simulink model "part_24"  (R2020a)
settings: Solver=FixedStepAuto  StartTime=0.0  StopTime=1000  FixedStep=0.1  RelTol=1e-3
values from neighbouring files (symbols this model uses):
  A_w = [zeros(3), eye(3) ... (first row only)    [init_NPO.m]
  C_w = [zeros(3) eye(3)]    [init_NPO.m]
  Cur_A_mu = 0.001    [init_current.m]
  Cur_Ac = 0    [init_current.m]
  D = [264860  0  0; 0  881640  0; 0  0  337740000]    [Kalman_data.mat]    (also in init_NPO.m = [2.6486e5  0         0)
  K1 = [diag([K_1i   K_1i   K_1i]) ... (first row only)    [init_NPO.m]
  K2 = K_2i * eye(3)    [init_NPO.m]
  K3 = 0.1*K4    [init_NPO.m]
  K4 = 100000*diag([1 1 100])    [init_NPO.m]
  M_inv = [1.46677031844e-07  0  0; 0  1.2695973473e-07  9.23036390732e-11; 0  9.23036390732e-11  2.80179152408e-10]    [Kalman_data.mat]    (also in init_NPO.m = inv(M))
  OB_mu = 0.001    [init_NPO.m]
  RM_Gamma_matrix = [RM_omega1^2 0 0; 0 RM_omega2^2 0; 0 0 RM_omega3^2]    [init_RM.m]
  RM_Omega_matrix = [2*RM_zeta1*RM_omega1 0 0; 0 2*RM_zeta2*RM_omega2 0; 0 0 2*RM_zeta3*RM_omega3]    [init_RM.m]
  RM_t1 = 15    [init_RM.m]
  RM_t2 = 15    [init_RM.m]
  RM_t3 = 15    [init_RM.m]
  setp_n = 6    [init_RM.m]
  setpoint = [0,0,0 ... (first row only)    [init_RM.m]
  T_b = diag([T_b1 T_b2 T_b3])    [init_NPO.m]
undefined symbols (not defined in the file or in its folder): DP_Kd_matrix, DP_Ki_matrix, DP_Kp_matrix, Hoerner, K, P_0, posX, posY, vessel, Wind_A_mu, Wind_Cw, Wind_mu, x_0
libraries: marine_gnc x9, simulink x5, marine_hydro x2
settings Model: OrderedModelArguments=off  Creator=jonbjor  LastModifiedBy=USER
settings DataIOCC: ReturnWorkspaceOutputs=off
settings DebuggingCC: ArithmeticOperatorsInVariantConditions=warning
settings SFSimCC: SimUseLocalCustomCode=off  CustomCodeUndefinedFunction=UseInterfaceOnly
settings RTWCC: RTWUseLocalCustomCode=off

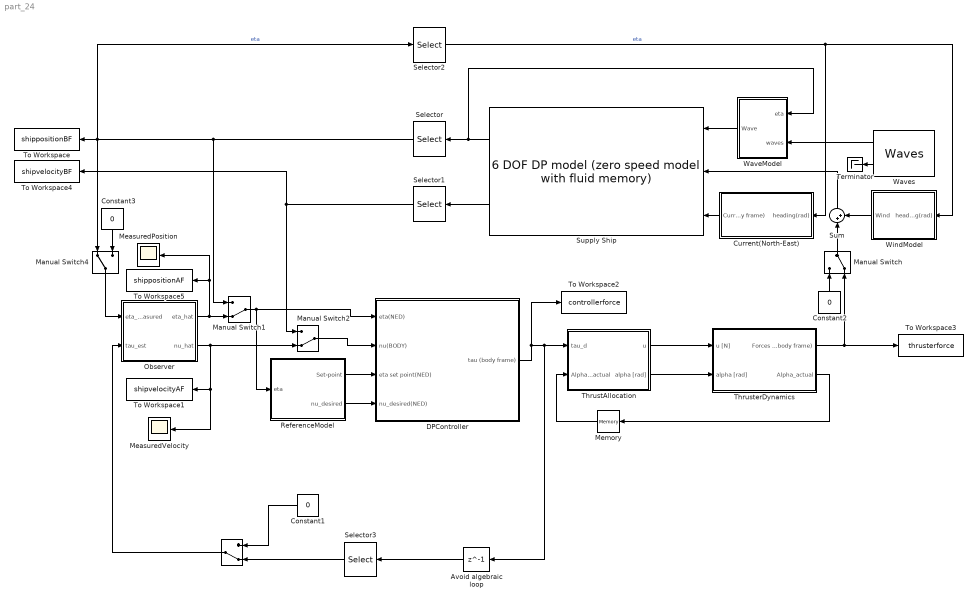
== system part_24 ==
  "\t\t" : ManualSwitch  CurrentSetting=0
  Avoid algebraic loop : Delay  DelayLength=1
  Constant1 : Constant  Value=0  VectorParams1D=off
  Constant2 : Constant  Value=0  VectorParams1D=off
  Constant3 : Constant  Value=0  VectorParams1D=off
  Current(North-East) : Subsystem
  DPController : Subsystem
  Manual Switch : ManualSwitch  CurrentSetting=0
  Manual Switch1 : ManualSwitch  CurrentSetting=0
  Manual Switch2 : ManualSwitch  CurrentSetting=0
  Manual Switch4 : ManualSwitch
  MeasuredPosition : Scope
  MeasuredVelocity : Scope
  Memory : Memory
  Observer : Subsystem
  ReferenceModel : Subsystem
  Selector : Selector  InputPortWidth=6  IndexOptions=Index vector (dialog)  Indices=[1 2 6]  OutputSizes=1
  Selector1 : Selector  InputPortWidth=6  IndexOptions=Index vector (dialog)  Indices=[1 2 6]  OutputSizes=1
  Selector2 : Selector  InputPortWidth=3  IndexOptions=Index vector (dialog)  Indices=[3]  OutputSizes=1
  Selector3 : Selector  InputPortWidth=6  IndexOptions=Index vector (dialog)  Indices=[1 2 6]  OutputSizes=1
  Sum : Sum  Inputs=|++
  Supply Ship : marine_hydro/Hydro Library/6 DOF DP model  (zero speed model with fluid memory)  ABC=vesselABC  rho=1025  Axc=0.9*vessel.main.T*vessel.main.B  Ayc=0.9*vessel.main.T*vessel.main.Lpp  CX=1  CY_2D=Hoerner(vessel.main.B,vessel.main.T)  Bv=vessel.Bv  mask(6 DOF zero speed model){}
      link override "Integrator1 ": InitialCondition=nu0
      link override Integrator2: InitialCondition=eta0
      settings: SourceProductName=MSS Hydro
      mask Display:
      | image('supply.jpg');
      | color('white'); port_label('output', 1, 'eta')
      | color('white'); port_label('output', 2, 'nu')
      | color('white'); port_label('input', 1, 'tau_wave')
      | color('white'); port_label('input', 2, 'tau')
      | color('white'); port_label('input', 3, 'nu_c')
  Terminator : Terminator
  ThrustAllocation : Subsystem
  ThrusterDynamics : Subsystem  mask{thrusterfault=off}
      mask prompts: thrusterfault "Fault on thruster #2 and #5?"
  To Workspace : ToWorkspace  VariableName=shippositionBF  SaveFormat=Structure With Time  SampleTime=-1
  To Workspace1 : ToWorkspace  VariableName=shipvelocityAF  SaveFormat=Structure With Time  SampleTime=-1
  To Workspace2 : ToWorkspace  VariableName=controllerforce  SaveFormat=Structure With Time  SampleTime=-1
  To Workspace3 : ToWorkspace  VariableName=thrusterforce  SaveFormat=Structure With Time  SampleTime=-1
  To Workspace4 : ToWorkspace  VariableName=shipvelocityBF  SaveFormat=Structure With Time  SampleTime=-1
  To Workspace5 : ToWorkspace  VariableName=shippositionAF  SaveFormat=Structure With Time  SampleTime=-1
  WaveModel : Subsystem  mask{waveforces=on}
      mask prompts: waveforces "Waveforces enabled"
  Waves : marine_gnc/Environment/Waves/Waves  spectrum_type=ITTC  disp_flag=on  plot_spectrum=off  plot_realization=off  hs=8  omega_peak=2*pi/13  psi_mean=5*pi/4  gamma=-1  spread=2  depth=inf  nfreq=20  ndir=10  energylim=0.005  freq_cutoff=3  dir_cutoff=0  rand_seed=123  rand_freq=off  rand_dir=off  Zeta_a=0  Omega=0  Phase=0  Wavenum=0  Psi=0
      settings: SourceProductName=MSS GNC
  WindModel : Subsystem
  wires:
  Supply Ship/2 -> Selector1/1
  ReferenceModel/1(Set-point) -> DPController/3(eta set point(NED))
  Supply Ship/1 -> WaveModel/1(eta), Selector/1
  Current(North-East)/1(Current(body frame)) -> Supply Ship/3
  WaveModel/1(Wave) -> Supply Ship/1
  Waves/1 -> WaveModel/2(waves)
  Waves/2 -> Terminator/1
  WindModel/1(Wind) -> Sum/2
  ThrusterDynamics/1("Forces (body frame) ") -> Manual Switch/2, To Workspace3/1
  Selector2/1 -> WindModel/1(heading(rad)), Current(North-East)/1(heading(rad))  "eta"
  ThrustAllocation/1(u) -> ThrusterDynamics/1(u [N])
  ThrustAllocation/2(alpha [rad]) -> ThrusterDynamics/2(alpha [rad])
  ReferenceModel/2(nu_desired) -> DPController/4(nu_desired(NED))
  Sum/1 -> Supply Ship/2
  Manual Switch/1 -> Sum/1
  Constant2/1 -> Manual Switch/1
  Memory/1 -> ThrustAllocation/2(Alpha_actual)
  ThrusterDynamics/2(Alpha_actual) -> Memory/1
  Selector/1 -> Manual Switch1/1, Selector2/1, To Workspace/1, Manual Switch4/1  "eta"
  Observer/2(nu_hat) -> MeasuredVelocity/1, To Workspace1/1, Manual Switch2/2
  Observer/1(eta_hat) -> MeasuredPosition/1, To Workspace5/1, Manual Switch1/2
  "\t\t"/1 -> Observer/2(tau_est)
  Constant1/1 -> "\t\t"/1
  Manual Switch4/1 -> Observer/1(eta_measured)
  Constant3/1 -> Manual Switch4/2
  Avoid algebraic loop/1 -> Selector3/1
  DPController/1(tau (body frame)) -> To Workspace2/1, Avoid algebraic loop/1, ThrustAllocation/1(tau_d)
  Manual Switch1/1 -> DPController/1(eta(NED)), ReferenceModel/1(eta)
  Manual Switch2/1 -> DPController/2(nu(BODY))
  Selector3/1 -> "\t\t"/2
  Selector1/1 -> To Workspace4/1, Manual Switch2/1

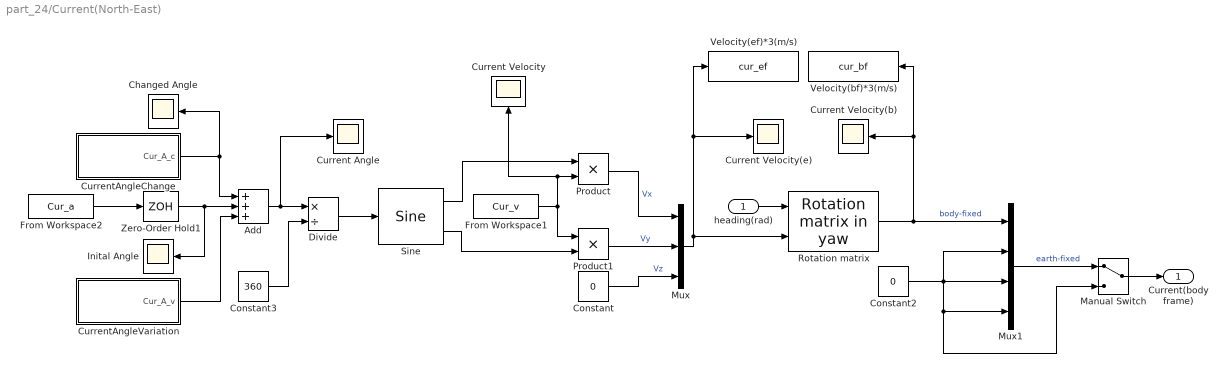
== system part_24/Current(North-East) ==
  heading(rad) : Inport
  Add : Sum  Inputs=+++
  Changed Angle : Scope
  Constant : Constant  Value=0
  Constant2 : Constant  Value=0  VectorParams1D=off
  Constant3 : Constant  Description=It is the angle of the current  Value=360
  Current Angle : Scope
  Current Velocity : Scope
  Current Velocity(b) : Scope
  Current Velocity(e) : Scope
  CurrentAngleChange : Subsystem
  CurrentAngleVariation : Subsystem
  Divide : Product  Inputs=*/
  From Workspace1 : FromWorkspace  VariableName=Cur_v  OutputAfterFinalValue=Holding final value
  From Workspace2 : FromWorkspace  VariableName=Cur_a  OutputAfterFinalValue=Holding final value
  Inital Angle : Scope
  Manual Switch : ManualSwitch
  Mux : Mux  Inputs=3
  Mux1 : Mux
  Product : Product
  Product1 : Product
  "Rotation matrix " : marine_gnc/Models/ Kinematics/Rotation matrix in yaw 
      settings: SourceProductName=MSS GNC
  Sine : simulink/Lookup Tables/Sine  Formula=sin(2*pi*u) and cos(2*pi*u)  NumDataPoints=(2^5)+1  OutputWordLength=16  InternalRulePriority=Speed
  Velocity(bf)*3(m/s) : ToWorkspace  VariableName=cur_bf  SaveFormat=Structure With Time  SampleTime=-1
  Velocity(ef)*3(m/s) : ToWorkspace  VariableName=cur_ef  SaveFormat=Structure With Time  SampleTime=-1
  Zero-Order Hold1 : ZeroOrderHold  SampleTime=-1
  Current(body frame) : Outport  VectorParamsAs1DForOutWhenUnconnected=off
  wires:
  From Workspace2/1 -> Zero-Order Hold1/1
  Sine/1 -> Product/1
  Divide/1 -> Sine/1
  Sine/2 -> Product1/2
  CurrentAngleChange/1(Cur_A_c) -> Add/1, Changed Angle/1
  From Workspace1/1 -> Current Velocity/1, Product/2, Product1/1
  Product/1 -> Mux/1  "Vx"
  Mux/1 -> Velocity(ef)*3(m/s)/1, Current Velocity(e)/1, "Rotation matrix "/2
  heading(rad)/1 -> "Rotation matrix "/1
  Product1/1 -> Mux/2  "Vy"
  "Rotation matrix "/1 -> Velocity(bf)*3(m/s)/1, Current Velocity(b)/1, Mux1/1  "body-fixed"
  Add/1 -> Current Angle/1, Divide/1
  Constant2/1 -> Mux1/2, Manual Switch/2, Mux1/4, Mux1/3
  Constant3/1 -> Divide/2
  Constant/1 -> Mux/3  "Vz"
  Manual Switch/1 -> Current(body frame)/1
  Zero-Order Hold1/1 -> Inital Angle/1, Add/2
  CurrentAngleVariation/1(Cur_A_v) -> Add/3
  Mux1/1 -> Manual Switch/1  "earth-fixed"

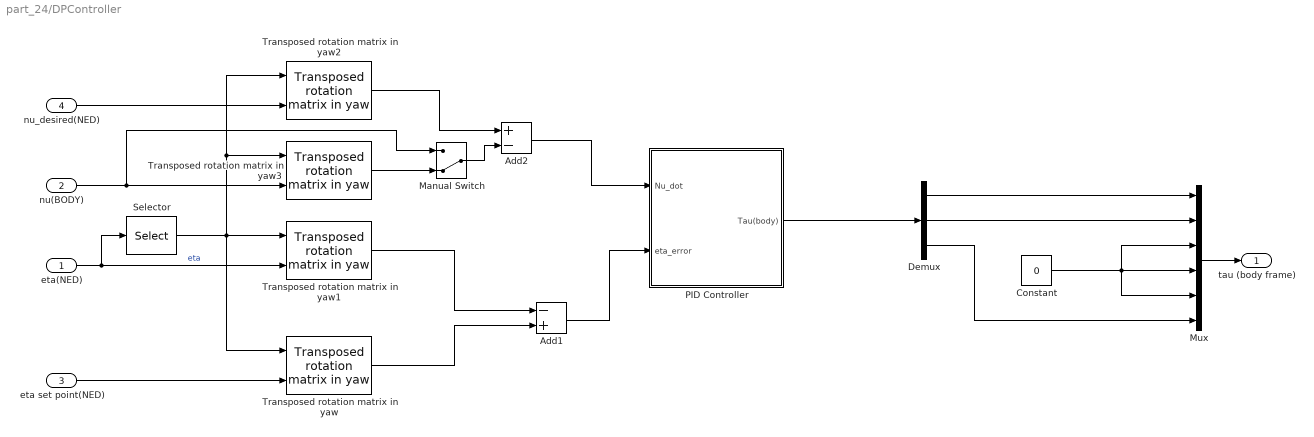
== system part_24/DPController ==
  eta(NED) : Inport
  nu(BODY) : Inport  Port=2
  eta set point(NED) : Inport  Port=3
  nu_desired(NED) : Inport  Port=4
  Add1 : Sum  Inputs=-+
  Add2 : Sum  Inputs=+-
  Constant : Constant  Value=0
  Demux : Demux  Outputs=3
  Manual Switch : ManualSwitch  CurrentSetting=0
  Mux : Mux  Inputs=6
  "PID Controller " : Subsystem
  Selector : Selector  InputPortWidth=3  IndexOptions=Starting index (dialog)  Indices=[3]  OutputSizes=1
  Transposed rotation matrix in yaw{,1..3} (4 alike) : marine_gnc/Models/ Kinematics/Transposed rotation  matrix in yaw
      settings: SourceProductName=MSS GNC
  tau (body frame) : Outport  VectorParamsAs1DForOutWhenUnconnected=off
  wires:
  nu_desired(NED)/1 -> Transposed rotation matrix in yaw2/2
  eta(NED)/1 -> Selector/1, Transposed rotation matrix in yaw1/2  "eta"
  Transposed rotation matrix in yaw1/1 -> Add1/1
  Transposed rotation matrix in yaw/1 -> Add1/2
  Add1/1 -> "PID Controller "/2("eta_error ")
  eta set point(NED)/1 -> Transposed rotation matrix in yaw/2
  "PID Controller "/1(Tau(body)) -> Demux/1
  Selector/1 -> Transposed rotation matrix in yaw3/1, Transposed rotation matrix in yaw2/1, Transposed rotation matrix in yaw/1, Transposed rotation matrix in yaw1/1
  Demux/2 -> Mux/2
  Add2/1 -> "PID Controller "/1("Nu_dot ")
  Demux/1 -> Mux/1
  Mux/1 -> tau (body frame)/1
  Transposed rotation matrix in yaw2/1 -> Add2/1
  Constant/1 -> Mux/5, Mux/4, Mux/3
  Demux/3 -> Mux/6
  Transposed rotation matrix in yaw3/1 -> Manual Switch/2
  Manual Switch/1 -> Add2/2
  nu(BODY)/1 -> Manual Switch/1, Transposed rotation matrix in yaw3/2

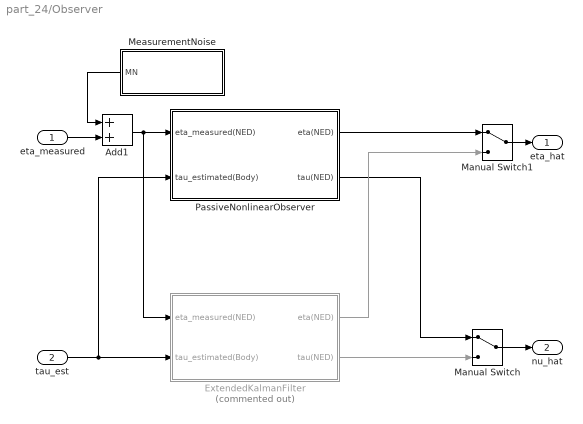
== system part_24/Observer ==
  eta_measured : Inport
  tau_est : Inport  Port=2
  Add1 : Sum
  ExtendedKalmanFilter : Subsystem  Commented=on
  Manual Switch : ManualSwitch
  Manual Switch1 : ManualSwitch
  MeasurementNoise : Subsystem
  PassiveNonlinearObserver : Subsystem
  eta_hat : Outport  VectorParamsAs1DForOutWhenUnconnected=off
  nu_hat : Outport  Port=2  VectorParamsAs1DForOutWhenUnconnected=off
  wires:
  PassiveNonlinearObserver/1(eta(NED)) -> Manual Switch1/1
  PassiveNonlinearObserver/2(tau(NED)) -> Manual Switch/1
  ExtendedKalmanFilter/1(eta(NED)) -> Manual Switch1/2
  ExtendedKalmanFilter/2(tau(NED)) -> Manual Switch/2
  tau_est/1 -> ExtendedKalmanFilter/2(tau_estimated(Body)), PassiveNonlinearObserver/2(tau_estimated(Body))
  Manual Switch/1 -> nu_hat/1
  Manual Switch1/1 -> eta_hat/1
  eta_measured/1 -> Add1/2
  Add1/1 -> ExtendedKalmanFilter/1(eta_measured(NED)), PassiveNonlinearObserver/1(eta_measured(NED))
  MeasurementNoise/1(MN) -> Add1/1

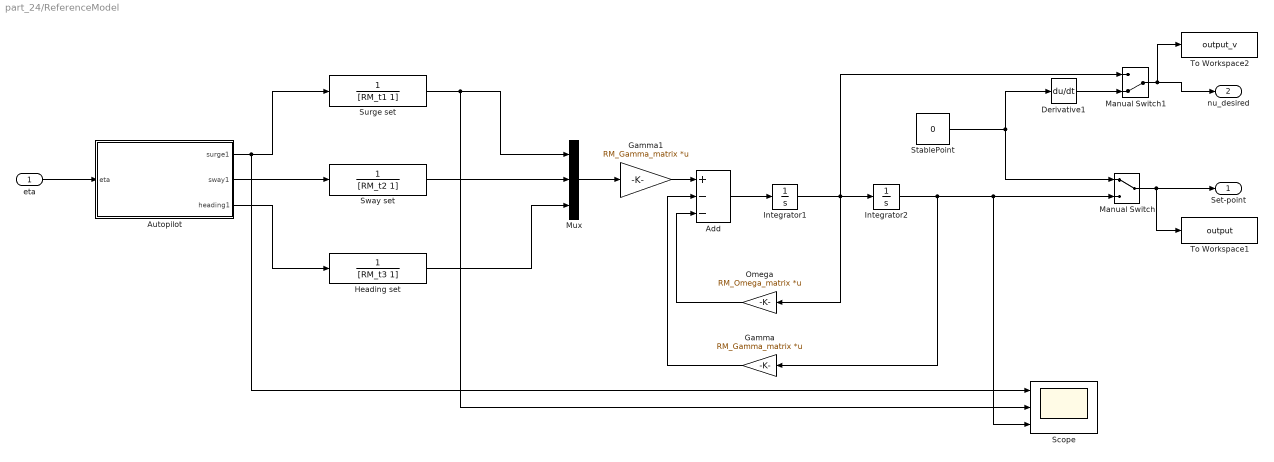
== system part_24/ReferenceModel ==
  eta : Inport
  Add : Sum  Inputs=+--
  Autopilot : Subsystem
  Derivative1 : Derivative
  Gamma : Gain  Gain=RM_Gamma_matrix  Multiplication=Matrix(K*u)
  Gamma1 : Gain  Gain=RM_Gamma_matrix  Multiplication=Matrix(K*u)
  Heading set : TransferFcn  Denominator=[RM_t3 1]
  Integrator1 : Integrator
  Integrator2 : Integrator
  Manual Switch : ManualSwitch
  Manual Switch1 : ManualSwitch  CurrentSetting=0
  Mux : Mux  Inputs=3
  Omega : Gain  Gain=RM_Omega_matrix  Multiplication=Matrix(K*u)
  Scope : Scope  NumInputPorts=3
  StablePoint : Constant  Value=0
  Surge set : TransferFcn  Denominator=[RM_t1 1]
  Sway set : TransferFcn  Denominator=[RM_t2 1]
  To Workspace1 : ToWorkspace  VariableName=output  SaveFormat=Structure With Time  SampleTime=-1
  To Workspace2 : ToWorkspace  VariableName=output_v  SaveFormat=Structure With Time  SampleTime=-1
  Set-point : Outport  VectorParamsAs1DForOutWhenUnconnected=off
  nu_desired : Outport  Port=2
  wires:
  Add/1 -> Integrator1/1
  StablePoint/1 -> Derivative1/1, Manual Switch/1
  Surge set/1 -> Mux/1, Scope/2
  Integrator1/1 -> Manual Switch1/1, Integrator2/1, Omega/1
  Gamma/1 -> Add/2
  Omega/1 -> Add/3
  Integrator2/1 -> Gamma/1, Scope/3, Manual Switch/2
  Heading set/1 -> Mux/3
  Mux/1 -> Gamma1/1
  Sway set/1 -> Mux/2
  Gamma1/1 -> Add/1
  Manual Switch/1 -> Set-point/1, To Workspace1/1
  eta/1 -> Autopilot/1(eta)
  Autopilot/1(surge1) -> Scope/1, Surge set/1
  Autopilot/2(sway1) -> Sway set/1
  Autopilot/3(heading1) -> Heading set/1
  Manual Switch1/1 -> To Workspace2/1, nu_desired/1
  Derivative1/1 -> Manual Switch1/2

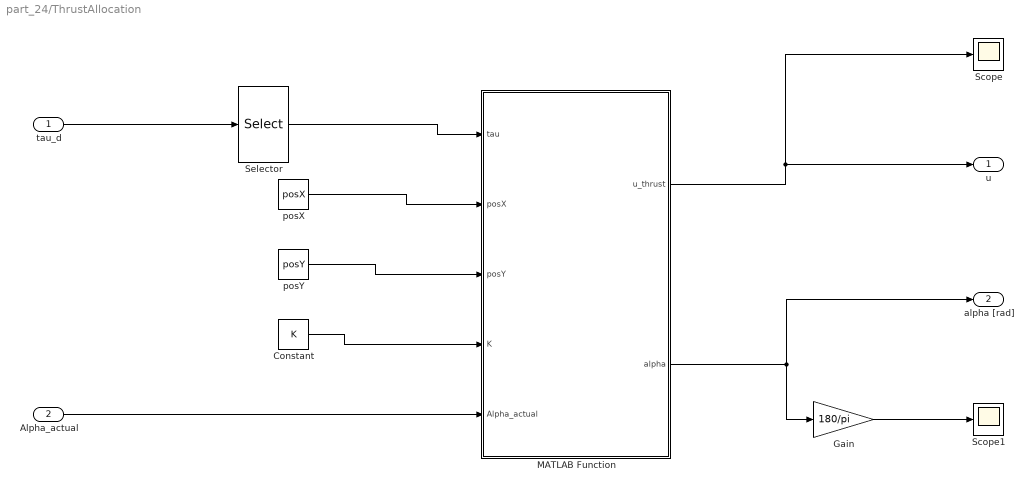
== system part_24/ThrustAllocation ==
  tau_d : Inport
  Alpha_actual : Inport  Port=2
  Constant : Constant  Value=K
  Gain : Gain  Gain=180/pi
  MATLAB Function : MATLAB Function  TreatAsAtomicUnit=on
  Scope : Scope
  Scope1 : Scope
  Selector : Selector  InputPortWidth=6  IndexOptions=Index vector (dialog)  Indices=[1 2 6 ]  OutputSizes=1
  posX : Constant  Value=posX
  posY : Constant  Value=posY
  u : Outport
  alpha [rad] : Outport  Port=2
  wires:
  tau_d/1 -> Selector/1
  MATLAB Function/1(u_thrust) -> Scope/1, u/1
  MATLAB Function/2(alpha) -> alpha [rad]/1, Gain/1
  Selector/1 -> MATLAB Function/1(tau)
  Gain/1 -> Scope1/1
  posX/1 -> MATLAB Function/2(posX)
  posY/1 -> MATLAB Function/3(posY)
  Constant/1 -> MATLAB Function/4(K)
  Alpha_actual/1 -> MATLAB Function/5(Alpha_actual)

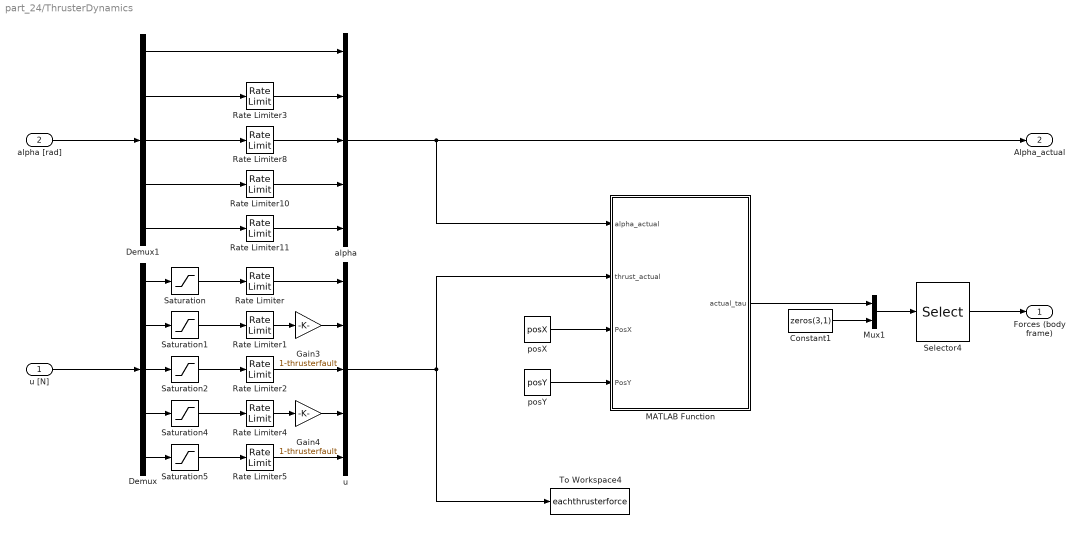
== system part_24/ThrusterDynamics ==
  u [N] : Inport
  alpha [rad] : Inport  Port=2
  Constant1 : Constant  Value=zeros(3,1)
  Demux : Demux  Outputs=5
  Demux1 : Demux  Outputs=5
  Gain3 : Gain  Gain=1-thrusterfault
  Gain4 : Gain  Gain=1-thrusterfault
  MATLAB Function : MATLAB Function  TreatAsAtomicUnit=on
  Mux1 : Mux  Inputs=2
  Rate Limiter : RateLimiter  RisingSlewLimit=15625  FallingSlewLimit=-15625  SampleTimeMode=inherited
  Rate Limiter1 : RateLimiter  RisingSlewLimit=18750  FallingSlewLimit=-18750  SampleTimeMode=inherited
  Rate Limiter{3,8,10..11} (4 alike) : RateLimiter  RisingSlewLimit=pi/15  FallingSlewLimit=-pi/15  SampleTimeMode=inherited
  Rate Limiter2 : RateLimiter  RisingSlewLimit=18750  FallingSlewLimit=-18750  SampleTimeMode=inherited
  Rate Limiter4 : RateLimiter  RisingSlewLimit=32000  FallingSlewLimit=-32000  SampleTimeMode=inherited
  Rate Limiter5 : RateLimiter  RisingSlewLimit=32000  FallingSlewLimit=-32000  SampleTimeMode=inherited
  Saturation : Saturate  UpperLimit=125000  LowerLimit=0
  Saturation1 : Saturate  UpperLimit=150000  LowerLimit=0
  Saturation2 : Saturate  UpperLimit=150000  LowerLimit=0
  Saturation4 : Saturate  UpperLimit=320000  LowerLimit=0
  Saturation5 : Saturate  UpperLimit=320000  LowerLimit=0
  Selector4 : Selector  InputPortWidth=6  IndexOptions=Index vector (dialog)  Indices=[1 2 4 5 6 3]  OutputSizes=1
  To Workspace4 : ToWorkspace  VariableName=eachthrusterforce  SaveFormat=Structure With Time  SampleTime=-1
  alpha : Mux  Inputs=5
  posX : Constant  Value=posX  VectorParams1D=off
  posY : Constant  Value=posY  VectorParams1D=off
  u : Mux  Inputs=5
  "Forces (body frame) " : Outport
  Alpha_actual : Outport  Port=2
  wires:
  Rate Limiter2/1 -> u/3
  Saturation/1 -> Rate Limiter/1
  Mux1/1 -> Selector4/1
  Constant1/1 -> Mux1/2
  Saturation4/1 -> Rate Limiter4/1
  Demux/2 -> Saturation1/1
  Saturation1/1 -> Rate Limiter1/1
  Demux/1 -> Saturation/1
  Demux/3 -> Saturation2/1
  Saturation2/1 -> Rate Limiter2/1
  Selector4/1 -> "Forces (body frame) "/1
  Rate Limiter/1 -> u/1
  Saturation5/1 -> Rate Limiter5/1
  Rate Limiter8/1 -> alpha/3
  u [N]/1 -> Demux/1
  alpha [rad]/1 -> Demux1/1
  posX/1 -> MATLAB Function/3(PosX)
  posY/1 -> MATLAB Function/4(PosY)
  alpha/1 -> Alpha_actual/1, MATLAB Function/1(alpha_actual)
  Demux1/3 -> Rate Limiter8/1
  Rate Limiter10/1 -> alpha/4
  Demux1/4 -> Rate Limiter10/1
  Demux1/5 -> Rate Limiter11/1
  Rate Limiter11/1 -> alpha/5
  Demux1/2 -> Rate Limiter3/1
  Demux1/1 -> alpha/1
  Demux/4 -> Saturation4/1
  Demux/5 -> Saturation5/1
  Rate Limiter5/1 -> u/5
  Rate Limiter3/1 -> alpha/2
  Rate Limiter1/1 -> Gain3/1
  MATLAB Function/1(actual_tau) -> Mux1/1
  u/1 -> To Workspace4/1, MATLAB Function/2(thrust_actual)
  Rate Limiter4/1 -> Gain4/1
  Gain3/1 -> u/2
  Gain4/1 -> u/4

== system part_24/WaveModel ==
  eta : Inport
  waves : Inport  Port=2
  Constant1 : Constant  Value=0  VectorParams1D=off
  Gain : Gain  Gain=waveforces
  Manual Switch1 : ManualSwitch  CurrentSetting=0
  Sum : Sum
  Wave loads (U=0) : marine_hydro/Hydro Library/Wave loads (U=0)  SystemSampleTime=-1  Latency=0  AutoFrameSizeCalculation=off
      settings: SourceProductName=MSS Hydro
  Wave : Outport  VectorParamsAs1DForOutWhenUnconnected=off
  wires:
  eta/1 -> Wave loads (U=0)/1
  waves/1 -> Wave loads (U=0)/2
  Sum/1 -> Gain/1
  Wave loads (U=0)/1 -> Sum/1
  Wave loads (U=0)/2 -> Sum/2
  Constant1/1 -> Manual Switch1/1
  Gain/1 -> Manual Switch1/2
  Manual Switch1/1 -> Wave/1

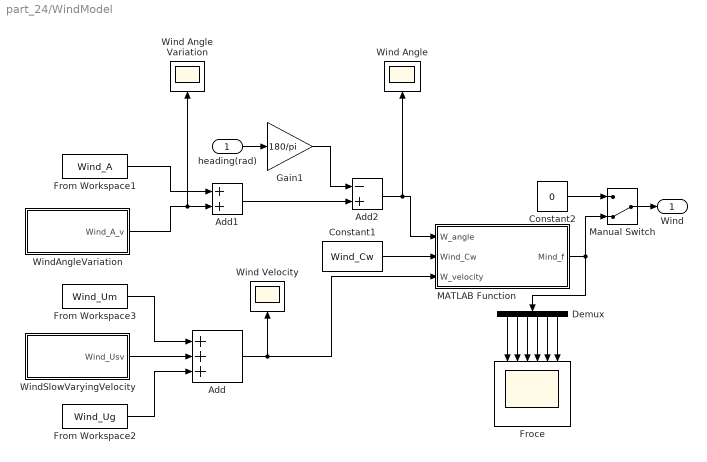
== system part_24/WindModel ==
  heading(rad) : Inport
  Add : Sum  Inputs=+++
  Add1 : Sum
  Add2 : Sum  Inputs=-+
  Constant1 : Constant  Value=Wind_Cw  SampleTime=0
  Constant2 : Constant  Value=0  VectorParams1D=off
  Demux : Demux  Outputs=6
  Froce : Scope  NumInputPorts=6
  From Workspace1 : FromWorkspace  VariableName=Wind_A  OutputAfterFinalValue=Holding final value
  From Workspace2 : FromWorkspace  VariableName=Wind_Ug  OutputAfterFinalValue=Holding final value
  From Workspace3 : FromWorkspace  VariableName=Wind_Um  OutputAfterFinalValue=Holding final value
  Gain1 : Gain  Gain=180/pi
  MATLAB Function : MATLAB Function  TreatAsAtomicUnit=on
  Manual Switch : ManualSwitch  CurrentSetting=0
  Wind Angle : Scope
  Wind Angle Variation : Scope
  Wind Velocity : Scope
  WindAngleVariation : Subsystem
  WindSlowVaryingVelocity : Subsystem
  Wind : Outport  VectorParamsAs1DForOutWhenUnconnected=off
  wires:
  Manual Switch/1 -> Wind/1
  From Workspace3/1 -> Add/1
  WindSlowVaryingVelocity/1(Wind_Usv) -> Add/2
  WindAngleVariation/1(Wind_A_v) -> Wind Angle Variation/1, Add1/2
  From Workspace1/1 -> Add1/1
  heading(rad)/1 -> Gain1/1
  Add1/1 -> Add2/2
  Gain1/1 -> Add2/1
  Add2/1 -> Wind Angle/1, MATLAB Function/1(W_angle)
  MATLAB Function/1(Mind_f) -> Manual Switch/2, Demux/1
  Constant1/1 -> MATLAB Function/2(Wind_Cw)
  Demux/1 -> Froce/1
  Demux/6 -> Froce/6
  Demux/5 -> Froce/5
  Demux/3 -> Froce/3
  Demux/2 -> Froce/2
  Demux/4 -> Froce/4
  Add/1 -> MATLAB Function/3(W_velocity), Wind Velocity/1
  From Workspace2/1 -> Add/3
  Constant2/1 -> Manual Switch/1

== system part_24/Current(North-East)/CurrentAngleChange ==
  Constant4 : Constant  Description=It is the angle of the current  Value=0
  Constant5 : Constant  Value=Cur_Ac
  From Workspace3 : FromWorkspace  VariableName=Cur_ac  SampleTime=0.1  Interpolate=off  OutputAfterFinalValue=Holding final value
  Switch : Switch  Criteria=u2 > Threshold
  Zero-Order Hold : ZeroOrderHold  SampleTime=-1
  Cur_A_c : Outport
  wires:
  Zero-Order Hold/1 -> Switch/1
  Constant5/1 -> Switch/2
  From Workspace3/1 -> Zero-Order Hold/1
  Constant4/1 -> Switch/3
  Switch/1 -> Cur_A_c/1

== system part_24/Current(North-East)/CurrentAngleVariation ==
  Add : Sum  Inputs=+-
  Band-Limited White Noise : simulink/Sources/Band-Limited White Noise  Cov=Cur_A_w  Ts=1  seed=[23341]
  Constant : Constant  Value=Cur_A_mu
  Integrator : Integrator
  prod : Product  Inputs=**
  Cur_A_v : Outport
  wires:
  Integrator/1 -> Cur_A_v/1, prod/2
  Constant/1 -> prod/1
  Band-Limited White Noise/1 -> Add/1
  prod/1 -> Add/2
  Add/1 -> Integrator/1  "Udot"

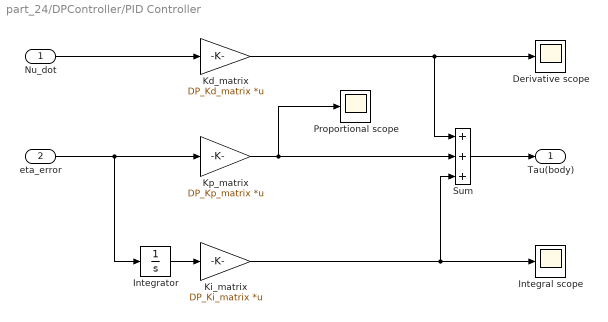
== system part_24/DPController/PID Controller  ==
  "Nu_dot " : Inport
  "eta_error " : Inport  Port=2
  "Derivative scope " : Scope
  "Integral scope " : Scope
  Integrator : Integrator
  "Kd_matrix " : Gain  Gain=DP_Kd_matrix  Multiplication=Matrix(K*u)
  "Ki_matrix " : Gain  Gain=DP_Ki_matrix  Multiplication=Matrix(K*u)
  Kp_matrix : Gain  Gain=DP_Kp_matrix  Multiplication=Matrix(K*u)
  "Proportional scope " : Scope
  Sum : Sum  Inputs=+++
  Tau(body) : Outport  VectorParamsAs1DForOutWhenUnconnected=off
  wires:
  "eta_error "/1 -> Integrator/1, Kp_matrix/1
  "Nu_dot "/1 -> "Kd_matrix "/1
  Integrator/1 -> "Ki_matrix "/1
  Kp_matrix/1 -> "Proportional scope "/1, Sum/2
  "Kd_matrix "/1 -> "Derivative scope "/1, Sum/1
  Sum/1 -> Tau(body)/1
  "Ki_matrix "/1 -> Sum/3, "Integral scope "/1

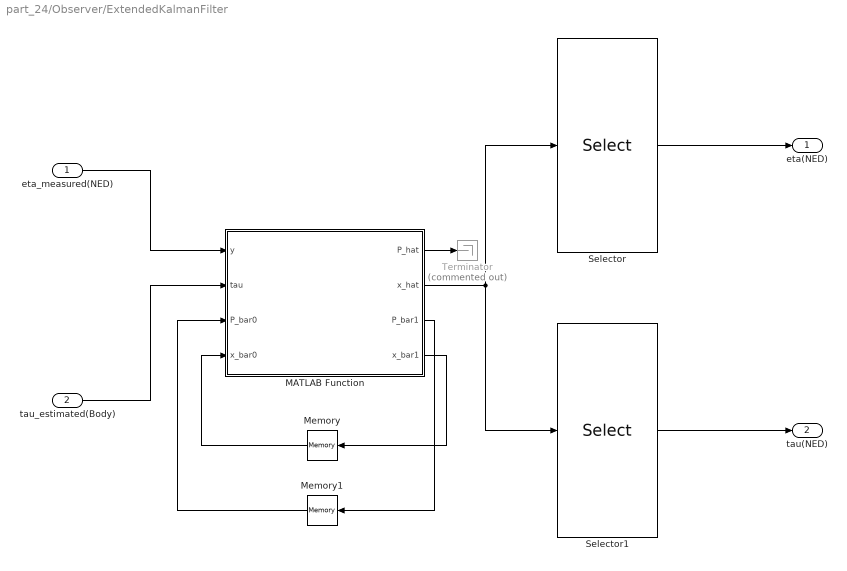
== system part_24/Observer/ExtendedKalmanFilter ==
  eta_measured(NED) : Inport
  tau_estimated(Body) : Inport  Port=2
  MATLAB Function : MATLAB Function  TreatAsAtomicUnit=on
  Memory : Memory  InitialCondition=x_0
  Memory1 : Memory  InitialCondition=P_0
  Selector : Selector  InputPortWidth=15  IndexOptions=Index vector (dialog)  Indices=[7 8 9]  OutputSizes=1
  Selector1 : Selector  InputPortWidth=15  IndexOptions=Index vector (dialog)  Indices=[13 14 15]  OutputSizes=1
  Terminator : Terminator  Commented=on
  eta(NED) : Outport
  tau(NED) : Outport  Port=2
  wires:
  eta_measured(NED)/1 -> MATLAB Function/1(y)
  tau_estimated(Body)/1 -> MATLAB Function/2(tau)
  Selector/1 -> eta(NED)/1
  Selector1/1 -> tau(NED)/1
  MATLAB Function/2(x_hat) -> Selector1/1, Selector/1
  MATLAB Function/1(P_hat) -> Terminator/1
  MATLAB Function/4(x_bar1) -> Memory/1
  Memory/1 -> MATLAB Function/4(x_bar0)
  MATLAB Function/3(P_bar1) -> Memory1/1
  Memory1/1 -> MATLAB Function/3(P_bar0)

== system part_24/Observer/MeasurementNoise ==
  Add : Sum  Inputs=+-
  Band-Limited White Noise : simulink/Sources/Band-Limited White Noise  Cov=OB_w  Ts=1  seed=[23341]
  Constant : Constant  Value=OB_mu
  Constant3 : Constant  Value=0  VectorParams1D=off
  Integrator : Integrator
  Manual Switch4 : ManualSwitch
  prod : Product  Inputs=**
  MN : Outport
  wires:
  Integrator/1 -> prod/2, Manual Switch4/2
  Constant/1 -> prod/1
  Band-Limited White Noise/1 -> Add/1
  prod/1 -> Add/2
  Add/1 -> Integrator/1  "Udot"
  Constant3/1 -> Manual Switch4/1
  Manual Switch4/1 -> MN/1

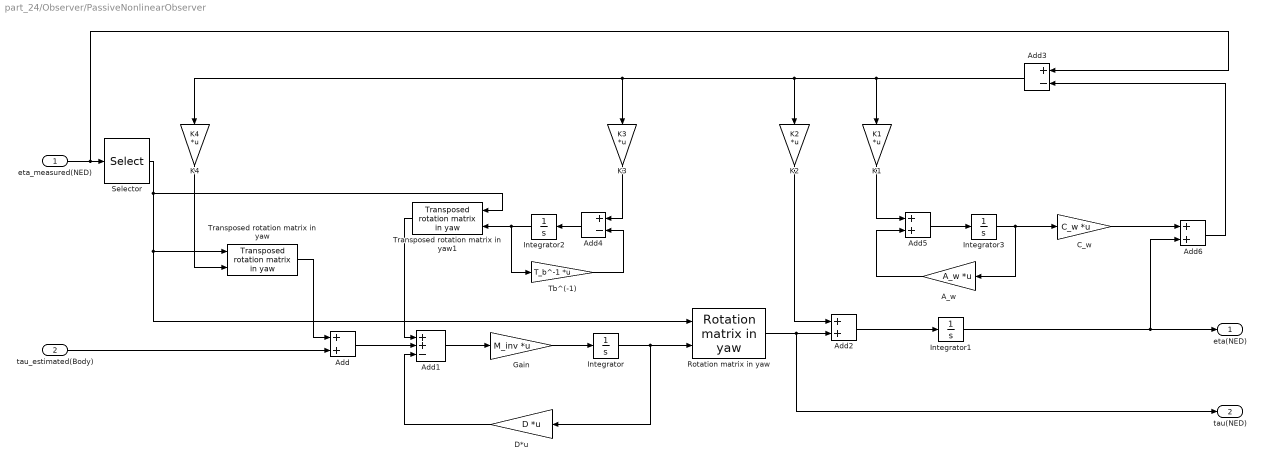
== system part_24/Observer/PassiveNonlinearObserver ==
  eta_measured(NED) : Inport
  tau_estimated(Body) : Inport  Port=2
  A_w : Gain  Gain=A_w  Multiplication=Matrix(K*u)
  Add{,2,5..6} (4 alike) : Sum
  Add1 : Sum  Inputs=++-
  Add3 : Sum  Inputs=+-
  Add4 : Sum  Inputs=+-
  C_w : Gain  Gain=C_w  Multiplication=Matrix(K*u)
  D*u : Gain  Gain=D  Multiplication=Matrix(K*u)
  Gain : Gain  Gain=M_inv  Multiplication=Matrix(K*u)
  Integrator{,1..3} (4 alike) : Integrator
  K1 : Gain  Gain=K1  Multiplication=Matrix(K*u)
  K2 : Gain  Gain=K2  Multiplication=Matrix(K*u)
  K3 : Gain  Gain=K3  Multiplication=Matrix(K*u)
  K4 : Gain  Gain=K4  Multiplication=Matrix(K*u)
  "Rotation matrix in yaw " : marine_gnc/Models/ Kinematics/Rotation matrix in yaw 
      settings: SourceProductName=MSS GNC
  Selector : Selector  InputPortWidth=3  IndexOptions=Index vector (dialog)  Indices=[3 ]  OutputSizes=1
  Tb^(-1) : Gain  Gain=T_b^-1  Multiplication=Matrix(K*u)
  Transposed rotation matrix in yaw : marine_gnc/Models/ Kinematics/Transposed rotation  matrix in yaw
      settings: SourceProductName=MSS GNC
  Transposed rotation matrix in yaw1 : marine_gnc/Models/ Kinematics/Transposed rotation  matrix in yaw
      settings: SourceProductName=MSS GNC
  eta(NED) : Outport
  tau(NED) : Outport  Port=2
  wires:
  eta_measured(NED)/1 -> Add3/1, Selector/1
  tau_estimated(Body)/1 -> Add/2
  Selector/1 -> "Rotation matrix in yaw "/1, Transposed rotation matrix in yaw/1, Transposed rotation matrix in yaw1/1
  Transposed rotation matrix in yaw/1 -> Add/1
  K4/1 -> Transposed rotation matrix in yaw/2
  Add/1 -> Add1/2
  Add1/1 -> Gain/1
  Gain/1 -> Integrator/1
  Integrator/1 -> D*u/1, "Rotation matrix in yaw "/2
  "Rotation matrix in yaw "/1 -> tau(NED)/1, Add2/2
  Add2/1 -> Integrator1/1
  Integrator1/1 -> Add6/2, eta(NED)/1
  Add3/1 -> K1/1, K2/1, K4/1, K3/1
  K2/1 -> Add2/1
  K3/1 -> Add4/1
  Add4/1 -> Integrator2/1
  Integrator2/1 -> Transposed rotation matrix in yaw1/2, Tb^(-1)/1
  Tb^(-1)/1 -> Add4/2
  Transposed rotation matrix in yaw1/1 -> Add1/1
  K1/1 -> Add5/1
  Add5/1 -> Integrator3/1
  A_w/1 -> Add5/2
  Integrator3/1 -> C_w/1, A_w/1
  C_w/1 -> Add6/1
  Add6/1 -> Add3/2
  D*u/1 -> Add1/3

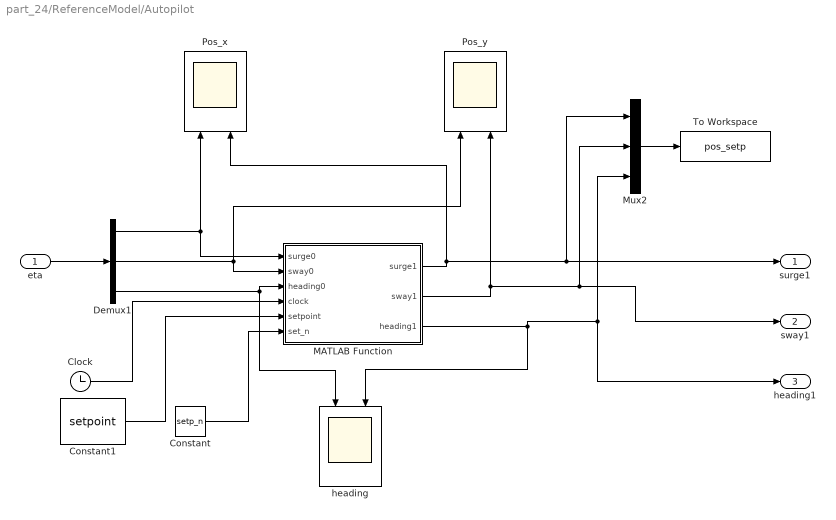
== system part_24/ReferenceModel/Autopilot ==
  eta : Inport
  Clock : Clock
  Constant : Constant  Value=setp_n
  Constant1 : Constant  Value=setpoint
  Demux1 : Demux  Outputs=3
  MATLAB Function : MATLAB Function  TreatAsAtomicUnit=on
  Mux2 : Mux  Inputs=3
  Pos_x : Scope  NumInputPorts=2
  Pos_y : Scope  NumInputPorts=2
  To Workspace : ToWorkspace  VariableName=pos_setp  SaveFormat=Structure With Time  SampleTime=-1
  heading : Scope  NumInputPorts=2
  surge1 : Outport
  sway1 : Outport  Port=2
  heading1 : Outport  Port=3
  wires:
  Mux2/1 -> To Workspace/1
  Demux1/3 -> heading/1, MATLAB Function/3(heading0)
  Demux1/2 -> MATLAB Function/2(sway0), Pos_y/1
  MATLAB Function/2(sway1) -> sway1/1, Mux2/2, Pos_y/2
  MATLAB Function/3(heading1) -> Mux2/3, heading1/1, heading/2
  eta/1 -> Demux1/1
  Demux1/1 -> MATLAB Function/1(surge0), Pos_x/1
  MATLAB Function/1(surge1) -> Pos_x/2, Mux2/1, surge1/1
  Constant/1 -> MATLAB Function/6(set_n)
  Constant1/1 -> MATLAB Function/5(setpoint)
  Clock/1 -> MATLAB Function/4(clock)

== system part_24/WindModel/WindAngleVariation ==
  Add : Sum  Inputs=+-
  Band-Limited White Noise : simulink/Sources/Band-Limited White Noise  Cov=Wind_A_w  Ts=1  seed=[23341]
  Constant : Constant  Value=Wind_A_mu
  Integrator : Integrator
  prod : Product  Inputs=**
  Wind_A_v : Outport
  wires:
  Integrator/1 -> Wind_A_v/1, prod/2
  Constant/1 -> prod/1
  Band-Limited White Noise/1 -> Add/1
  prod/1 -> Add/2
  Add/1 -> Integrator/1  "Udot"

== system part_24/WindModel/WindSlowVaryingVelocity ==
  Add : Sum  Inputs=+-
  Band-Limited White Noise : simulink/Sources/Band-Limited White Noise  Cov=Wind_w  Ts=1  seed=[23341]
  Constant : Constant  Value=Wind_mu
  Integrator : Integrator
  prod : Product  Inputs=**
  Wind_Usv : Outport
  wires:
  Integrator/1 -> Wind_Usv/1, prod/2
  Constant/1 -> prod/1
  Band-Limited White Noise/1 -> Add/1
  prod/1 -> Add/2
  Add/1 -> Integrator/1  "Udot"

== matlab function part_24/ThrustAllocation/MATLAB Function ==
  data: tau input; u_thrust output; posX input; posY input; K input; alpha output; Alpha_actual input

function [u_thrust , alpha] = extended_thrust_allocation(tau,posX,posY,K,Alpha_actual)


T_extended = [0,1,0,1,0,1,0,1,0;1,0,1,0,1,0,1,0,1;
    posX(1),0,posY(2),0,posX(3),posY(4),posX(4),posY(5),posX(5)];

% thruster angles
u_e = inv(K)*pinv(T_extended)*tau;

u_thrust_2 = sqrt(u_e(2)^2 + u_e(3)^2);
u_thrust_3 = sqrt(u_e(4)^2 + u_e(5)^2);
u_thrust_4 = sqrt(u_e(6)^2 + u_e(7)^2);
u_thrust_5 = sqrt(u_e(8)^2 + u_e(9)^2);

u_thrust = [u_e(1);u_thrust_2;u_thrust_3;u_thrust_4;u_thrust_5];
 
% alpha
alpha = zeros(5,1);
alpha(1) = pi/2;
alpha(2) = atan2(u_e(3),u_e(2));
alpha(3) = atan2(u_e(5),u_e(4));
alpha(4) = atan2(u_e(7),u_e(6));
alpha(5) = atan2(u_e(9),u_e(8));

%Limiting thrust to azimuths under heavy position change
for i = 2:5
    if(alpha(i) > Alpha_actual(i) + 10*pi/180 || alpha(i) < Alpha_actual(i) - 10*pi/180)
        u_thrust(i) = 0;
    end
end


% checking forbidden sectors:
if alpha(4) > pi/4 && alpha(4,1) <= 3*pi/8
    alpha(4) = pi/4;
elseif alpha(4) > 3*pi/8 && alpha(4) < pi/2
    alpha(4) = pi/2;
end

if alpha(5) > -pi/4 && alpha(4,1) <= -3*pi/8
    alpha(5) = -pi/4;
elseif alpha(5) > -3*pi/8 && alpha(5) < -pi/2
    alpha(5) = -pi/2;
end

end

== matlab function part_24/WindModel/MATLAB Function ==
  data: W_angle input; Wind_Cw input; Mind_f output; W_velocity input
function Mind_f = fcn(W_angle,Wind_Cw, W_velocity)
W_cw=zeros(6,1);

%Set judgement=[0,360)
if W_angle<0
    judgement=W_angle+360;
elseif W_angle>=360
    judgement=W_angle-360;
    else
        judgement=W_angle;
end

%do judgement
w1=0;       %weighting of angles
w2=0;
for i=1:36
    if judgement>=Wind_Cw(i,1) && judgement<Wind_Cw(i+1,1)
        w1=1-(judgement-Wind_Cw(i,1))/10;
        w2=(judgement-Wind_Cw(i,1))/10;
        W_cw(1)=w1*Wind_Cw(i,2)+w2*Wind_Cw(i+1,2);    %force
        W_cw(2)=w1*Wind_Cw(i,3)+w2*Wind_Cw(i+1,3);
        W_cw(3)=w1*Wind_Cw(i,4)+w2*Wind_Cw(i+1,4);
        W_cw(4)=w1*Wind_Cw(i,5)+w2*Wind_Cw(i+1,5);    %moment
        W_cw(5)=w1*Wind_Cw(i,6)+w2*Wind_Cw(i+1,6);
        W_cw(6)=w1*Wind_Cw(i,7)+w2*Wind_Cw(i+1,7);
    end
end
Mind_force = abs(W_velocity)^2 * W_cw';
Mind_f = Mind_force';
end

== matlab function part_24/Observer/ExtendedKalmanFilter/MATLAB Function ==
  settings: updateMethod=DISCRETE  sampleTime=0.1
  data: P_hat output; y input; tau input; x_hat output; P_bar0 input; x_bar0 input; P_bar1 output; x_bar1 output
function [P_hat, x_hat, P_bar1, x_bar1] = ExtendedKalmanFilter(y, tau, P_bar0, x_bar0)

persistent Aw B_kf H_kf E_kf M_inv D...
     R_kf Q_kf... 
    h_step Tb Phi 

Data = load('Kalman_data.mat');

   [Aw,B_kf,H_kf,E_kf,R_kf,Q_kf, M_inv, D, ~, ~, h_step, Tb] = ...
        deal(Data.Aw, Data.B, Data.H, Data.E,...
        Data.R,Data.Q,Data.M_inv,Data.D,Data.Zetan,...
        Data.Wn, Data.Ts, Data.Tb);


%Computing kalman gain based on prediction
K = (P_bar0*H_kf')/((H_kf*P_bar0*H_kf' + R_kf));

%Update the error covariance matrix with prediction estimate
P_hat = (eye(15) - K*H_kf)*P_bar0*(eye(15)-K*H_kf)' + K*R_kf*K';

%Correction: Update predicted estimate with measurement
x_hat = x_bar0 + K*(y-H_kf*x_bar0);

%Linearization
Phi = eye(15) + h_step*Jacobi(x_hat, Aw, Tb,M_inv,D);
gamma = h_step*E_kf;

%Prediction
P_bar1 = Phi*P_hat*Phi' + gamma*Q_kf*gamma';
x_bar1 = x_hat + h_step*(f(x_hat,Aw,Tb,M_inv,D) + B_kf*tau);

% x =[xi_1 til x_6, N(7), E(8), psi(9),b1(10), b2(11), b3(12), u(13),
% v(14),r(15)], n=15 states
end

%% Jacobi
function [J] = Jacobi(x_hat, Aw, Tb, M_inv, D)
J = [Aw zeros(6,9);zeros(9,15)];
% J(1,:) = [0 0 0 1 0 0    0 0 0      0 0 0       0 0 0];
% J(2,:) = [0 0 0 0 1 0    0 0 0      0 0 0       0 0 0];
% J(3,:) = [0 0 0 0 0 1    0 0 0      0 0 0       0 0 0];
% J(4,:) = [-(Wn(1))^2-2*Zetan(1)*Wn(1) 0 0      0 0 0   0 0 0   0 0 0   0 0 0];
% J(5,:) = [0 -(Wn(2))^2-2*Zetan(2)*Wn(2) 0      0 0 0   0 0 0   0 0 0   0 0 0];
% J(6,:) = [0 0 -(Wn(3))^2-2*Zetan(3)*Wn(3)      0 0 0   0 0 0   0 0 0   0 0 0];

J(7,:) = [0 0 0 0 0 0   0 0 -sin(x_hat(9))*x_hat(13)-cos(x_hat(9))*x_hat(14)     0 0 0   cos(x_hat(9)) -sin(x_hat(9)) 0]; 
J(8,:) = [0 0 0 0 0 0   0 0 cos(x_hat(9))*x_hat(13)-sin(x_hat(9))*x_hat(14)      0 0 0   sin(x_hat(9)) cos(x_hat(9))  0];
J(9,:) = [0 0 0 0 0 0   0 0 0                           0 0 0   0 0 1];

J(10,:) = [0 0 0 0 0 0  0 0 0   inv(-Tb(1)) 0 0    0 0 0];
J(11,:) = [0 0 0 0 0 0  0 0 0   0 inv(-Tb(2)) 0    0 0 0];
J(12,:) = [0 0 0 0 0 0  0 0 0   0 0 inv(-Tb(3))    0 0 0];

J(13,:) = [0 0 0 0 0 0  0 0 M_inv(1,1)*(-sin(x_hat(9))*x_hat(10)+cos(x_hat(9))*x_hat(11))   M_inv(1,1)*cos(x_hat(9)) M_inv(1,1)*sin(x_hat(9)) 0               -M_inv(1,1)*D(1,1) 0 0];
J(14,:) = [0 0 0 0 0 0  0 0 M_inv(2,2)*(-cos(x_hat(9))*x_hat(10)-sin(x_hat(9))*x_hat(11))   M_inv(2,2)*sin(x_hat(9)) M_inv(2,2)*cos(x_hat(9)) M_inv(2,3)      0 -M_inv(2,2)*D(2,2) -M_inv(2,3)*D(3,3)];
J(15,:) = [0 0 0 0 0 0  0 0 M_inv(3,2)*(-cos(x_hat(9))*x_hat(10)-cos(x_hat(9))*x_hat(11))   M_inv(3,2)*(-sin(x_hat(9))) M_inv(3,2)*cos(x_hat(9)) M_inv(3,3)    0 M_inv(3,2) M_inv(3,3)*D(3,3)];
 end
                          

function f = f(x_hat, Aw, Tb, M_inv, D)
    Tb_inv = (Tb).^(-1);

    f = zeros(15,1);
    f(1:6,1) = Aw*x_hat(1:6,1);
    f(7:9,1) = R(x_hat(9,1))*x_hat(13:15,1);
    f(10:12,1) = -(Tb_inv)*x_hat(10:12,1);
    f(13:15,1) = (-M_inv*D*x_hat(13:15,1))...
    + M_inv*(R(x_hat(9,1)))'*x_hat(10:12,1);
end

function Rotation = R(psi)
     Rotation = [cos(psi) -sin(psi) 0;
            sin(psi) cos(psi) 0;
            0   0   1];
end

== matlab function part_24/ThrusterDynamics/MATLAB Function ==
  data: alpha_actual input; thrust_actual input; actual_tau output; PosX input; PosY input
function actual_tau   = fcn(alpha_actual,thrust_actual,PosX,PosY)

    Alpha_surge =[cos(alpha_actual(1)) cos(alpha_actual(2)) cos(alpha_actual(3)) cos(alpha_actual(4)) cos(alpha_actual(5))];  
    Alpha_sway = [sin(alpha_actual(1)) sin(alpha_actual(2)) sin(alpha_actual(3)) sin(alpha_actual(4)) sin(alpha_actual(5))];
    Alpha_yaw = [sin(alpha_actual(1))*PosX(1)-cos(alpha_actual(1))*PosY(1) sin(alpha_actual(2))*PosX(2)-cos(alpha_actual(2))*PosY(2) ...
                 sin(alpha_actual(3))*PosX(3)-cos(alpha_actual(3))*PosY(3) sin(alpha_actual(4))*PosX(4)-cos(alpha_actual(4))*PosY(4) ...
                 sin(alpha_actual(5))*PosX(5)-cos(alpha_actual(5))*PosY(5)];

    actual_tau = [Alpha_surge; Alpha_sway; Alpha_yaw]*thrust_actual;
end

== matlab function part_24/ReferenceModel/Autopilot/MATLAB Function ==
  settings: updateMethod=DISCRETE
  data: surge1 output; sway1 output; surge0 input; sway0 input; heading0 input; clock input; heading1 output; setpoint input; set_n input
function [surge1, sway1, heading1] = fcn(surge0, sway0, heading0, clock, setpoint, set_n)
persistent stv
if isempty(stv) 
    stv=1;
end
%触发器
persistent trigger
if isempty(trigger) 
    trigger = 0;
end
%start time
persistent starttime
if isempty(starttime) 
    starttime = 0;
end


j=set_n;                                %judgement value of setpoint
k=0.1;                                  %judgement value
duration = 30;                          %The duration time(30s)

surge1 = setpoint(stv,1);
sway1 = setpoint(stv,2);
heading1 = setpoint(stv,3);

if trigger == 0
    %the ship is closed to the set point
    if abs(surge0-surge1)<k && abs(sway0-sway1)<k && abs(heading0-heading1)<k*0.05
        starttime = clock;
        trigger = 1;
    end
end

if trigger == 1
    if clock - starttime > duration
        %after duration, ship is stable
        if stv<j                              %we have not reached the final setpoint
            if abs(surge0-surge1)<k && abs(sway0-sway1)<k && abs(heading0-heading1)<k*0.05
                stv=stv+1;
                surge1=setpoint(stv,1);
                sway1=setpoint(stv,2);
                heading1=setpoint(stv,3);
                trigger = 0;
            end
        end        
    end
end
end
